simulink model "sampleModel1982_sub_sub"  (R2023a)
settings: Solver=VariableStepAuto  StartTime=0.0  StopTime=10.0  RelTol=1e-3
libraries: hdlsllib x5, simulink x1
settings Model: Creator=user1  LastModifiedBy=user1
settings OptimizationCC: BlockReduction=off  ConditionallyExecuteInputs=off

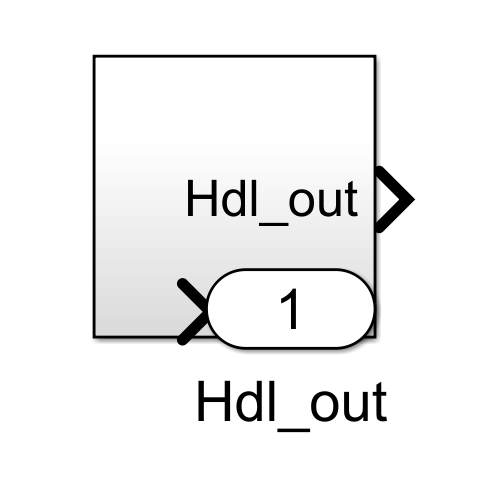
[thumbnail: Simulink's stored preview of the top-level diagram]
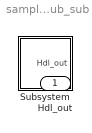
== system sampleModel1982_sub_sub ==
  Subsystem : Subsystem
  Hdl_out : Outport  OutDataTypeStr=uint8

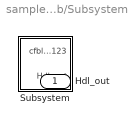
== system sampleModel1982_sub_sub/Subsystem ==
  Subsystem : Subsystem
  Hdl_out : Outport  OutDataTypeStr=uint8

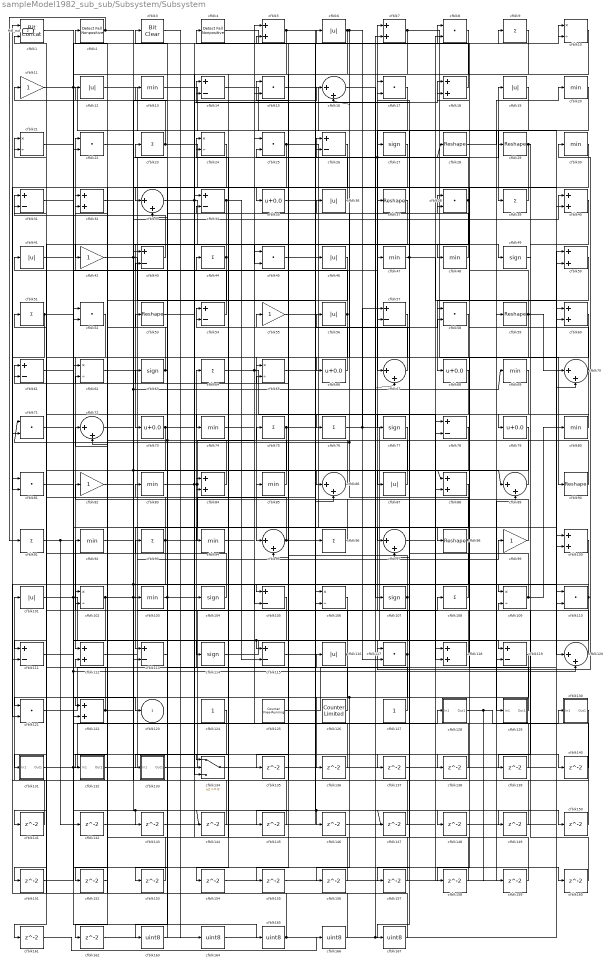
== system sampleModel1982_sub_sub/Subsystem/Subsystem ==
  cfblk1 : hdlsllib/Logic and Bit Operations/Bit Concat  numInputs=2
  cfblk{10,21,24,62,65,102,106,109} (8 alike) : Product  Inputs=*/  OutDataTypeStr=uint8  RndMeth=Zero  SaturateOnIntegerOverflow=on
  cfblk{5,7,18,32,40,50,60,84,88,100,112,118,122} (13 alike) : Sum  OutDataTypeStr=uint8
  cfblk{6,12,19,36,41,46,56,87,101,116} (10 alike) : Abs  OutDataTypeStr=uint8  SaturateOnIntegerOverflow=off
  cfblk{13,20,30,47..48,69,74,80,83,85,92,94,103} (13 alike) : MinMax  OutDataTypeStr=uint8
  cfblk{27,49,63,77,104,107,114} (7 alike) : Signum
  cfblk{14,26,31,34,43,54,57,61,78,105,111,113,115,119} (14 alike) : Sum  Inputs=+-  OutDataTypeStr=uint8
  cfblk{9,23,39,44,51,64,75..76,91,93,96,108} (12 alike) : Sum  Inputs=+  OutDataTypeStr=uint8
  cfblk{11,42,55,82,99} (5 alike) : Gain  OutDataTypeStr=uint8
  cfblk{8,15,17,22,25,38,45,52,58,71,81,110,117,121} (14 alike) : DotProduct  OutDataTypeStr=uint8
  cfblk{16,33,67,70,72,86,89,95,97,120} (10 alike) : Sum  Inputs=|++  OutDataTypeStr=uint8
  cfblk124 : Constant  OutDataTypeStr=uint8  SampleTime=-1
  cfblk125 : hdlsllib/Sources/Counter Free-Running  NumBits=16  tsamp=-1
  cfblk126 : hdlsllib/Sources/Counter Limited  uplimit=7  tsamp=-1
  cfblk127 : Constant  OutDataTypeStr=uint8  SampleTime=-1
  cfblk128 : Subsystem
      settings: LibrarySourceBlock=|
      | hdlsllib/Ports &
      | Subsystems/Subsystem
  cfblk129 : Subsystem
      settings: LibrarySourceBlock=|
      | hdlsllib/Ports &
      | Subsystems/Subsystem
  cfblk130 : Subsystem
      settings: LibrarySourceBlock=|
      | hdlsllib/Ports &
      | Subsystems/Subsystem
  cfblk131 : Subsystem
      settings: LibrarySourceBlock=|
      | hdlsllib/Ports &
      | Subsystems/Subsystem
  cfblk132 : Subsystem
      settings: LibrarySourceBlock=|
      | hdlsllib/Ports &
      | Subsystems/Subsystem
  cfblk133 : Subsystem
      settings: LibrarySourceBlock=|
      | hdlsllib/Ports &
      | Subsystems/Subsystem
  cfblk134 : Switch  OutDataTypeStr=uint8  SaturateOnIntegerOverflow=off  InputSameDT=off
  cfblk{135..162} (28 alike) : Delay  SampleTime=1
  cfblk{163..167} (5 alike) : DataTypeConversion  OutDataTypeStr=uint8  SaturateOnIntegerOverflow=off  RndMeth=Floor
  cfblk2 : hdlsllib/Logic and Bit Operations/Detect Fall Nonpositive  vinit=0  OutDataTypeStr=uint8
  cfblk{28..29,37,53,59,90,98} (7 alike) : Reshape
  cfblk3 : simulink/Logic and Bit Operations/Bit Clear  iBit=0
      settings: LibrarySourceBlock=|
      | hdlsllib/Logic and Bit
      | Operations/Bit Clear
  cfblk{35,66,68,73,79} (5 alike) : Bias  Bias=0.0  SaturateOnIntegerOverflow=off
  cfblk4 : hdlsllib/Logic and Bit Operations/Detect Fall Nonpositive  vinit=0  OutDataTypeStr=uint8
  cfblk123 : Outport  OutDataTypeStr=uint8  VectorParamsAs1DForOutWhenUnconnected=off
  Hdl_out : Outport  Port=2  OutDataTypeStr=uint8
  wires:
  cfblk167/1 -> cfblk1/2
  cfblk137/1 -> cfblk167/1
  cfblk166/1 -> cfblk1/1
  cfblk161/1 -> cfblk166/1
  cfblk165/1 -> cfblk60/1, cfblk62/2
  cfblk164/1 -> cfblk70/2, cfblk67/2
  cfblk163/1 -> cfblk3/1
  cfblk124/1 -> cfblk163/1
  cfblk162/1 -> cfblk7/2
  cfblk37/1 -> cfblk161/1
  cfblk160/1 -> cfblk109/2
  cfblk159/1 -> cfblk97/2
  cfblk158/1 -> cfblk72/1
  cfblk60/1 -> cfblk158/1
  cfblk157/1 -> cfblk34/1
  cfblk156/1 -> cfblk24/2
  cfblk155/1 -> cfblk8/2
  cfblk154/1 -> cfblk89/2
  cfblk153/1 -> cfblk32/2
  cfblk152/1 -> cfblk102/2
  cfblk151/1 -> cfblk22/2
  cfblk57/1 -> cfblk151/1
  cfblk150/1 -> cfblk17/2
  cfblk149/1 -> cfblk5/2
  cfblk148/1 -> cfblk50/2
  cfblk147/1 -> cfblk84/2
  cfblk146/1 -> cfblk78/1
  cfblk145/1 -> cfblk54/2
  cfblk26/1 -> cfblk145/1
  cfblk144/1 -> cfblk43/1
  cfblk143/1 -> cfblk33/2
  cfblk142/1 -> cfblk86/2
  cfblk141/1 -> cfblk81/1
  cfblk140/1 -> cfblk52/1
  cfblk111/1 -> cfblk140/1
  cfblk139/1 -> cfblk62/1
  cfblk40/1 -> cfblk139/1
  cfblk138/1 -> cfblk45/1
  cfblk92/1 -> cfblk138/1
  cfblk136/1 -> cfblk112/2
  cfblk135/1 -> cfblk65/2
  cfblk106/1 -> cfblk135/1
  cfblk45/1 -> cfblk78/2
  cfblk2/1 -> cfblk91/1, cfblk40/2
  cfblk113/1 -> cfblk93/1
  cfblk82/1 -> cfblk40/1, cfblk89/1
  cfblk20/1 -> cfblk77/1
  cfblk59/1 -> cfblk111/1, cfblk70/1, cfblk38/2
  cfblk81/1 -> cfblk6/1
  cfblk49/1 -> cfblk109/1
  cfblk96/1 -> cfblk84/1
  cfblk129/1(Out1) -> cfblk38/1
  cfblk125/1 -> cfblk100/1
  cfblk78/1 -> cfblk134/1
  cfblk87/1 -> cfblk13/1, cfblk41/1
  cfblk107/1 -> cfblk115/1, cfblk132/1(In1), cfblk61/1
  cfblk24/1 -> cfblk81/2
  cfblk5/1 -> cfblk106/1, cfblk52/2
  cfblk54/1 -> cfblk32/1
  cfblk73/1 -> cfblk110/2, cfblk131/1(In1)
  cfblk41/1 -> cfblk114/1
  cfblk119/1 -> cfblk155/1, cfblk156/1
  cfblk21/1 -> cfblk117/1
  cfblk28/1 -> cfblk20/1
  cfblk22/1 -> cfblk105/2, cfblk150/1, cfblk88/2
  cfblk1/1 -> cfblk165/1
  cfblk32/1 -> cfblk48/1
  cfblk74/1 -> cfblk15/2
  cfblk116/1 -> cfblk63/1, cfblk141/1
  cfblk84/1 -> cfblk11/1
  cfblk104/1 -> cfblk21/1
  cfblk15/1 -> cfblk110/1
  cfblk122/1 -> cfblk14/2, cfblk69/1, cfblk21/2
  cfblk110/1 -> cfblk105/1, cfblk113/2
  cfblk42/1 -> cfblk88/1, cfblk134/3, cfblk96/1
  cfblk103/1 -> cfblk53/1, cfblk17/1
  cfblk90/1 -> cfblk8/1
  cfblk23/1 -> cfblk59/1, cfblk12/1
  cfblk14/1 -> cfblk26/2
  cfblk36/1 -> cfblk15/1
  cfblk61/1 -> cfblk120/2, cfblk137/1
  cfblk30/1 -> cfblk72/2
  cfblk93/1 -> cfblk31/2, cfblk111/2, cfblk57/2
  cfblk16/1 -> cfblk107/1
  cfblk133/1(Out1) -> cfblk5/1
  cfblk85/1 -> cfblk34/2
  cfblk80/1 -> cfblk76/1
  cfblk19/1 -> cfblk97/1
  cfblk101/1 -> cfblk119/2, cfblk47/1
  cfblk134/1 -> cfblk50/1
  cfblk13/1 -> cfblk120/1
  cfblk72/1 -> cfblk86/1
  cfblk31/1 -> cfblk143/1, cfblk144/1
  cfblk64/1 -> cfblk118/2, cfblk18/2
  cfblk68/1 -> cfblk103/1
  cfblk34/1 -> cfblk73/1, cfblk115/2
  cfblk91/1 -> cfblk123/1, cfblk142/1
  cfblk95/1 -> cfblk51/1, cfblk149/1
  cfblk27/1 -> cfblk37/1
  cfblk43/1 -> cfblk31/1
  cfblk63/1 -> cfblk2/1, cfblk43/2
  cfblk131/1(Out1) -> cfblk128/1(In1), cfblk160/1
  cfblk3/1 -> cfblk164/1
  cfblk65/1 -> cfblk46/1
  cfblk71/1 -> cfblk146/1, cfblk147/1
  cfblk6/1 -> cfblk117/2, cfblk16/2, cfblk35/1
  cfblk7/1 -> cfblk90/1, cfblk134/2
  cfblk8/1 -> cfblk65/1
  cfblk10/1 -> cfblk66/1
  cfblk86/1 -> cfblk75/1
  cfblk39/1 -> cfblk33/1
  cfblk55/1 -> cfblk29/1
  cfblk38/1 -> cfblk25/2, cfblk154/1
  cfblk127/1 -> cfblk83/1
  cfblk66/1 -> cfblk56/1
  cfblk100/1 -> cfblk121/2
  cfblk70/1 -> cfblk121/1, cfblk18/1
  cfblk67/1 -> cfblk24/1
  cfblk83/1 -> cfblk25/1, cfblk100/2, cfblk9/1
  cfblk130/1(Out1) -> cfblk101/1
  cfblk46/1 -> cfblk133/1(In1)
  cfblk102/1 -> cfblk28/1, cfblk27/1, cfblk99/1, cfblk122/2
  cfblk4/1 -> cfblk10/2
  cfblk115/1 -> cfblk10/1
  cfblk51/1 -> cfblk71/2, cfblk148/1
  cfblk99/1 -> cfblk82/1
  cfblk109/1 -> cfblk55/1, cfblk80/1
  cfblk69/1 -> cfblk95/2
  cfblk35/1 -> cfblk49/1
  cfblk29/1 -> cfblk79/1, cfblk58/1
  cfblk33/1 -> cfblk45/2, cfblk16/1
  cfblk128/1(Out1) -> cfblk130/1(In1), cfblk159/1
  cfblk12/1 -> cfblk129/1(In1)
  cfblk98/1 -> cfblk71/1, cfblk36/1, cfblk152/1
  cfblk117/1 -> cfblk61/2, cfblk136/1
  cfblk79/1 -> cfblk87/1
  cfblk105/1 -> cfblk122/1
  cfblk50/1 -> cfblk68/1
  cfblk97/1 -> cfblk118/1
  cfblk94/1 -> cfblk26/1
  cfblk53/1 -> cfblk104/1
  cfblk88/1 -> cfblk113/1
  cfblk77/1 -> cfblk85/1
  cfblk18/1 -> cfblk4/1
  cfblk9/1 -> cfblk74/1
  cfblk47/1 -> cfblk60/2, cfblk157/1
  cfblk58/1 -> cfblk95/1
  cfblk108/1 -> cfblk14/1
  cfblk114/1 -> cfblk30/1
  cfblk76/1 -> cfblk119/1, cfblk57/1
  cfblk44/1 -> cfblk42/1, cfblk162/1
  cfblk25/1 -> cfblk98/1, cfblk153/1
  cfblk112/1 -> cfblk44/1
  cfblk11/1 -> cfblk39/1, cfblk94/1
  cfblk75/1 -> cfblk102/1, cfblk58/2
  cfblk132/1(Out1) -> cfblk108/1
  cfblk121/1 -> cfblk116/1
  cfblk89/1 -> cfblk54/1
  cfblk62/1 -> cfblk19/1
  cfblk48/1 -> cfblk23/1
  cfblk126/1 -> cfblk64/1
  cfblk17/1 -> cfblk67/1
  cfblk120/1 -> cfblk92/1
  cfblk118/1 -> cfblk7/1
  cfblk56/1 -> cfblk22/1, cfblk106/2
  cfblk52/1 -> cfblk112/1

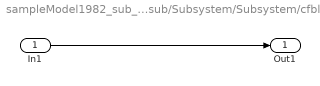
== system sampleModel1982_sub_sub/Subsystem/Subsystem/cfblk128 ==
  In1 : Inport
  Out1 : Outport
  wires:
  In1/1 -> Out1/1

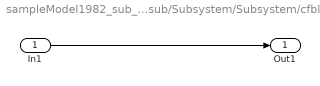
== system sampleModel1982_sub_sub/Subsystem/Subsystem/cfblk129 ==
  In1 : Inport
  Out1 : Outport
  wires:
  In1/1 -> Out1/1

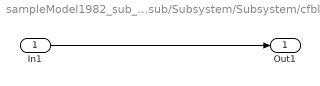
== system sampleModel1982_sub_sub/Subsystem/Subsystem/cfblk130 ==
  In1 : Inport
  Out1 : Outport
  wires:
  In1/1 -> Out1/1

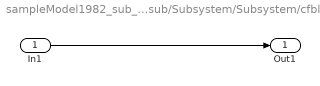
== system sampleModel1982_sub_sub/Subsystem/Subsystem/cfblk131 ==
  In1 : Inport
  Out1 : Outport
  wires:
  In1/1 -> Out1/1

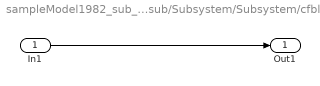
== system sampleModel1982_sub_sub/Subsystem/Subsystem/cfblk132 ==
  In1 : Inport
  Out1 : Outport
  wires:
  In1/1 -> Out1/1

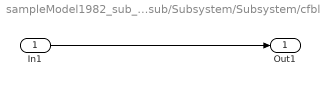
== system sampleModel1982_sub_sub/Subsystem/Subsystem/cfblk133 ==
  In1 : Inport
  Out1 : Outport
  wires:
  In1/1 -> Out1/1
